simulink model "q_qube2_bal_rl_hw"  (R2021a)
settings: Solver=ode1  StartTime=0.0  StopTime=inf  FixedStep=Ts  RelTol=1e-3  EnableMultiTasking=on
undefined symbols (not defined in the file or in its folder): alpha_bal_threshold, HIL, qc_get_step_size
libraries: quarc_library x3, simulink_extras x2, deeplib x1, simulink x1
settings Model: SimulationMode=external  ExtModeTrigDuration=10000  Creator=MLevis  LastModifiedBy=MLevis
settings SolverCC: AlgebraicLoopSolver=TrustRegion  PositivePriorityOrder=on
settings DataIOCC: ReturnWorkspaceOutputs=off
settings DebuggingCC: UnderspecifiedInitializationDetection=Classic  MergeDetectMultiDrivingBlocksExec=none  SFMachineParentedDataDiag=warning
settings ModelReferenceCC: PropagateSignalLabelsOutOfModel=off
settings SFSimCC: CustomCodeUndefinedFunction=UseInterfaceOnly
settings RTWCC: Description=QUARC Win64 Target Using Toolchain  SystemTargetFile=quarc_win64.tlc  TemplateMakefile=quarc_default_tmf  Toolchain=QUARC win64 | nmake (64-bit Windows)  BuildConfiguration=Faster Runs
settings STFCustomTargetCC: TargetLangStandard=C99 (ISO)  ConcurrentExecutionCompliant=on  SystemTargetFile=quarc_win64.tlc
settings GRTTargetCC: ParMdlRefBuildCompliant=off  CompOptLevelCompliant=off  CombineOutputUpdateFcns=off  MatFileLogging=off  CPPClassGenCompliant=off  GRTInterface=on  ExtMode=on  ExtModeMexFile=quarc_comm

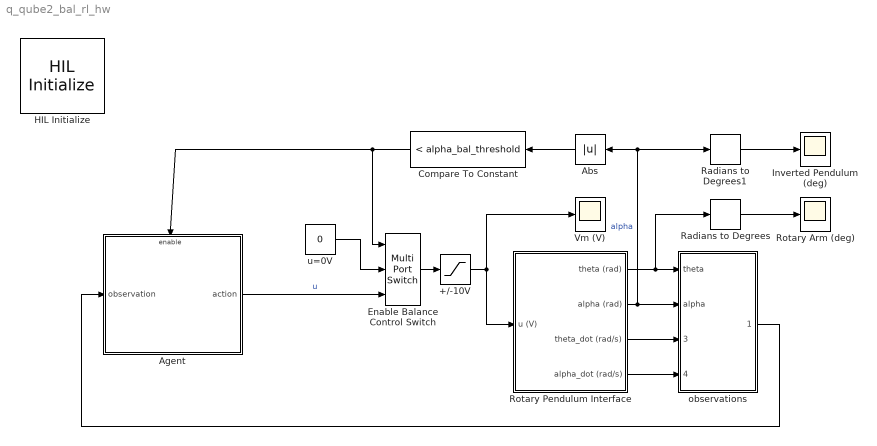
== system q_qube2_bal_rl_hw ==
  +/-10V : Saturate  UpperLimit=10  LowerLimit=-10
  Abs : Abs
  Agent : Subsystem
  Compare To Constant : simulink/Logic and Bit Operations/Compare To Constant  relop=<  const=alpha_bal_threshold  OutDataTypeStr=boolean
  Enable Balance Control Switch : MultiPortSwitch  DataPortOrder=Zero-based contiguous  Inputs=2  zeroidx=on
  HIL Initialize : quarc_library/Data Acquisition/Generic/Configuration/HIL Initialize  object_name=HIL-1  board_type=qube_servo2_usb  board_number=0  board_options=""  exclusive=off  active=on  hardware_clocks=[0]  clock_modes=[]  initial_clock_frequencies=[]  set_clock_params_at_start=off  set_clock_params_at_switch_in=off  set_clock_frequencies_at_start=off  set_clock_frequencies_at_switch_in=off  analog_input_channels=[0]  analog_input_configurations=[]  analog_input_maximums=3  analog_input_minimums=-3  set_analog_input_params_at_start=off  set_analog_input_params_at_switch_in=off  analog_output_channels=[0]  analog_output_maximums=15  analog_output_minimums=-15  initial_analog_outputs=[0]  final_analog_outputs=[0]  watchdog_analog_outputs=0  set_analog_output_params_at_start=off  set_analog_output_params_at_switch_in=off  set_analog_outputs_at_start=on  set_analog_outputs_at_switch_in=off  set_analog_outputs_at_terminate=on  set_analog_outputs_at_switch_out=off  set_analog_outputs_on_watchdog=on  digital_input_channels=[]  digital_output_channels=[0]  digital_output_configuration=[]  initial_digital_outputs=[1]  final_digital_outputs=[0]  watchdog_digital_outputs=[0]  set_digital_output_params_at_start=off  set_digital_output_params_at_switch_in=off  set_digital_outputs_at_start=on  set_digital_outputs_at_switch_in=off  set_digital_outputs_at_terminate=on  set_digital_outputs_at_switch_out=off  set_digital_outputs_on_watchdog=on  encoder_channels=[0:1]  quadrature=[4]  encoder_filter_frequency=[]  initial_encoder_counts=[0]  set_encoder_params_at_start=off  set_encoder_params_at_switch_in=off  set_encoder_counts_at_start=on  set_encoder_counts_at_switch_in=off  pwm_channels=[]  pwm_modes=[]  pwm_frequency=[]  pwm_configuration=[]  pwm_alignment=[]  pwm_polarity=[]  pwm_leading_deadband=[]  pwm_trailing_deadband=[]  initial_pwm_outputs=[]  final_pwm_outputs=[]  watchdog_pwm_outputs=[]  set_pwm_params_at_start=off  set_pwm_params_at_switch_in=off  set_pwm_outputs_at_start=off  set_pwm_outputs_at_switch_in=off  set_pwm_outputs_at_terminate=off  set_pwm_outputs_at_switch_out=off  set_pwm_outputs_on_watchdog=off  other_output_channels=[11000:11002]  initial_other_outputs=[0 1 0]  final_other_outputs=[1 0 0]  watchdog_other_outputs=[0 0 1]  set_other_outputs_at_start=on  set_other_outputs_at_switch_in=off  set_other_outputs_at_terminate=on  set_other_outputs_at_switch_out=off  set_other_outputs_on_watchdog=on
  Inverted Pendulum (deg) : Scope
  Radians to Degrees : simulink_extras/Transformations/Radians to Degrees
  Radians to Degrees1 : simulink_extras/Transformations/Radians to Degrees
  Rotary Arm (deg) : Scope
  Rotary Pendulum Interface : Subsystem
  Vm (V) : Scope
  observations : Subsystem  VariantControl=sincos
  u=0V : Constant  Value=0
  wires:
  Radians to Degrees/1 -> Rotary Arm (deg)/1
  Radians to Degrees1/1 -> Inverted Pendulum (deg)/1
  +/-10V/1 -> Rotary Pendulum Interface/1(u (V)), Vm (V)/1
  Rotary Pendulum Interface/1(theta (rad)) -> observations/1(theta), Radians to Degrees/1
  Rotary Pendulum Interface/3(theta_dot (rad/s)) -> observations/3(theta_dot)
  Rotary Pendulum Interface/4(alpha_dot (rad/s)) -> observations/4(alpha_dot)
  observations/1(observations) -> Agent/1(observation)
  Compare To Constant/1 -> Agent/Enable, Enable Balance Control Switch/1
  Rotary Pendulum Interface/2(alpha (rad)) -> Radians to Degrees1/1, Abs/1, observations/2(alpha)  "alpha"
  Abs/1 -> Compare To Constant/1
  Enable Balance Control Switch/1 -> +/-10V/1
  u=0V/1 -> Enable Balance Control Switch/2
  Agent/1(action) -> Enable Balance Control Switch/3  "u"

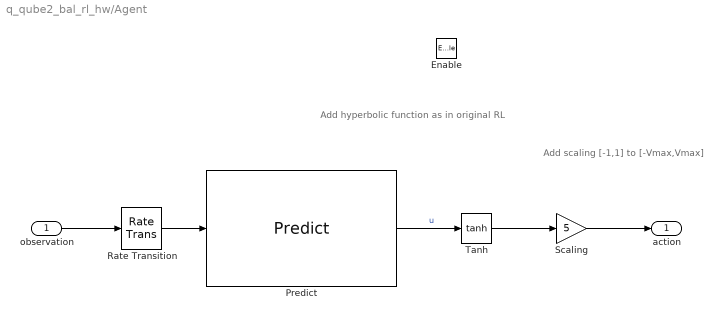
== system q_qube2_bal_rl_hw/Agent ==
  note: Add hyperbolic function as in original RL
  note: Add scaling [-1,1] to [-Vmax,Vmax]
  observation : Inport
  Enable : EnablePort
  Predict : deeplib/Predict  Network=Network from MAT-file  NetworkFunction=squeezenet  NetworkFilePath=D:\Documents\Current_Dev\QUBE_IP_Bal_Release_R2021a\QubeIPBalRLPolicy.mat  MiniBatchSize=128  InputDataFormats={ '', '' }  Predictions=on  Activations={}  ForceInterpretedSim=off  EnableDLNetwork=on
      settings: SourceProductBaseCode=NN
  Rate Transition : RateTransition
  Scaling : Gain  Gain=5
  Tanh : Trigonometry  Operator=tanh
  action : Outport  InitialOutput=[0]
  wires:
  observation/1 -> Rate Transition/1
  Predict/1 -> Tanh/1  "u"
  Tanh/1 -> Scaling/1
  Scaling/1 -> action/1
  Rate Transition/1 -> Predict/1

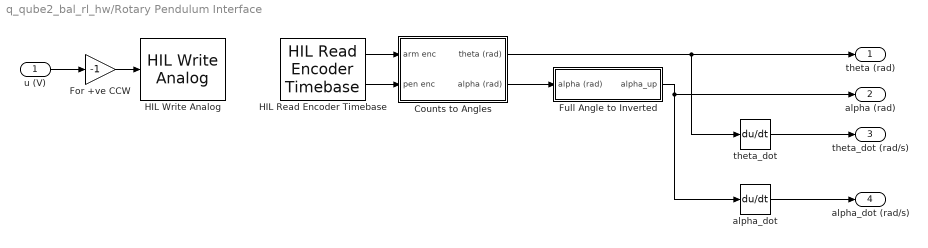
== system q_qube2_bal_rl_hw/Rotary Pendulum Interface ==
  u (V) : Inport
  Counts to Angles : Subsystem
  For +ve CCW : Gain  Gain=-1
  Full Angle to Inverted : Subsystem
  HIL Read Encoder Timebase : quarc_library/Data Acquisition/Generic/Timebases/HIL Read Encoder Timebase  object_name=HIL-1  clock=0  channels=[0:1]  active=on  vector_output=off  data_type_mode=Inherit via back propagation  data_type=double  overflow_mode=Error on overflow  samples_in_buffer=max(ceil(1/qc_get_step_size), 1)
  HIL Write Analog : quarc_library/Data Acquisition/Generic/Immediate I//O/HIL Write Analog  object_name=HIL-1  channels=0  sample_time=-1  active=on  vector_input=off
  alpha_dot : Derivative
  theta_dot : Derivative
  theta (rad) : Outport  VectorParamsAs1DForOutWhenUnconnected=off
  alpha (rad) : Outport  Port=2  VectorParamsAs1DForOutWhenUnconnected=off
  theta_dot (rad/s) : Outport  Port=3  VectorParamsAs1DForOutWhenUnconnected=off
  alpha_dot (rad/s) : Outport  Port=4  VectorParamsAs1DForOutWhenUnconnected=off
  wires:
  For +ve CCW/1 -> HIL Write Analog/1
  u (V)/1 -> For +ve CCW/1
  HIL Read Encoder Timebase/1 -> Counts to Angles/1(arm enc)
  HIL Read Encoder Timebase/2 -> Counts to Angles/2(pen enc)
  Counts to Angles/1(theta (rad)) -> theta (rad)/1, theta_dot/1
  Counts to Angles/2(alpha (rad)) -> Full Angle to Inverted/1(alpha (rad))
  Full Angle to Inverted/1(alpha_up) -> alpha (rad)/1, alpha_dot/1
  alpha_dot/1 -> alpha_dot (rad/s)/1
  theta_dot/1 -> theta_dot (rad/s)/1

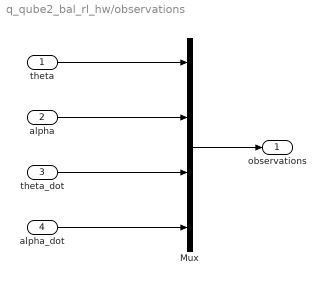
== system q_qube2_bal_rl_hw/observations ==
  theta : Inport
  alpha : Inport  Port=2
  theta_dot : Inport  Port=3
  alpha_dot : Inport  Port=4
  Mux : Mux
  observations : Outport  VectorParamsAs1DForOutWhenUnconnected=off
  wires:
  alpha_dot/1 -> Mux/4
  theta_dot/1 -> Mux/3
  alpha/1 -> Mux/2
  theta/1 -> Mux/1
  Mux/1 -> observations/1

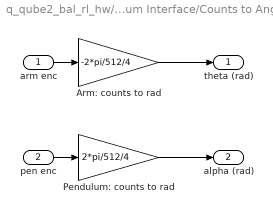
== system q_qube2_bal_rl_hw/Rotary Pendulum Interface/Counts to Angles ==
  arm enc : Inport
  pen enc : Inport  Port=2
  Arm: counts to rad : Gain  Gain=-2*pi/512/4
  Pendulum: counts to rad : Gain  Gain=2*pi/512/4
  theta (rad) : Outport  VectorParamsAs1DForOutWhenUnconnected=off
  alpha (rad) : Outport  Port=2  VectorParamsAs1DForOutWhenUnconnected=off
  wires:
  pen enc/1 -> Pendulum: counts to rad/1
  arm enc/1 -> Arm: counts to rad/1
  Arm: counts to rad/1 -> theta (rad)/1
  Pendulum: counts to rad/1 -> alpha (rad)/1

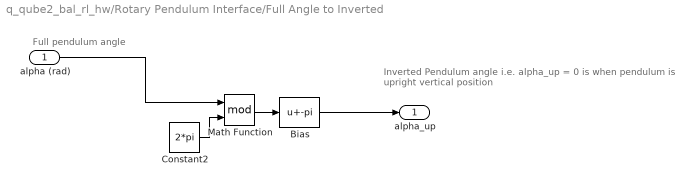
== system q_qube2_bal_rl_hw/Rotary Pendulum Interface/Full Angle to Inverted ==
  note: Full pendulum angle
  note: Inverted Pendulum angle
      | i.e. alpha_up = 0 is when pendulum is upright vertical position
  alpha (rad) : Inport
  Bias : Bias  Bias=-pi
  Constant2 : Constant  Value=2*pi
  Math Function : Math  Operator=mod  SignedPower=on  SaturateOnIntegerOverflow=on
  alpha_up : Outport  VectorParamsAs1DForOutWhenUnconnected=off
  wires:
  Math Function/1 -> Bias/1
  alpha (rad)/1 -> Math Function/1
  Bias/1 -> alpha_up/1
  Constant2/1 -> Math Function/2
